simulink model "sm_vehicle_2axle_heave_roll_grid"  (R2024a)
settings: Solver=ode23t  StartTime=0.0  StopTime=14.2  MaxStep=0.2  RelTol=1e-3  AbsTol=1e-3  EnableMultiTasking=on
PostLoadFcn:
  | sm_vehicle_2axle_heave_roll_param
  | sm_vehicle_2axle_heave_roll_scene
  | sm_vehicle_2axle_heave_roll_config_maneuver(bdroot,VehicleData,'rough road');
StartFcn:
  | tic
StopFcn:
  | Elapsed_Sim_Time = toc;
undefined symbols (not defined in the file): InitVehicle, Maneuver, SceneData, VehicleData, X, Y, Z
libraries: sm_lib x48, sm_vehicle_utilities_lib x13, nesl_utility x11
(part 1 of 2)
CloseFcn:
  | try,close(h1_sm_vehicle_2axle_heave_roll),end
  | clear h1_sm_vehicle_2axle_heave_roll
  | try,close(h2_sm_vehicle_2axle_heave_roll),end
  | clear h2_sm_vehicle_2axle_heave_roll
  | try,close(h3_sm_vehicle_2axle_heave_roll),end
  | clear h3_sm_vehicle_2axle_heave_roll
  | 
  | 
  | clear simlog_sm_vehicle_2axle_heave_roll
  | clear logsout_sm_vehicle_2axle_heave_roll
Description:
  | Vehicle Dynamics, 14 DOF Model, Uneven Terrain
  | 
  | Copyright 2022-2024 The MathWorks, Inc.
settings Model: Creator=smiller  LastModifiedBy=smiller
settings SolverCC: AutoScaleAbsTol=off  AlgebraicLoopSolver=TrustRegion
settings DataIOCC: SaveFormat=Array  SaveOutput=off  ReturnWorkspaceOutputs=off  SignalLoggingName=logsout_sm_vehicle_2axle_heave_roll_grid  OutputTimes=[0:0.01:10]
settings OptimizationCC: ReuseModelBlockBuffer=off  ExpressionDepthLimit=2147483647  LifeSpan=inf
settings DebuggingCC: UnderspecifiedInitializationDetection=Classic  MergeDetectMultiDrivingBlocksExec=none  SolverPrmCheckMsg=warning  UnconnectedInputMsg=warning  UnconnectedOutputMsg=warning  UnconnectedLineMsg=warning  StateNameClashWarn=warning  PregeneratedLibrarySubsystemCodeDiagnostic=none  SFUnexpectedBacktrackingDiag=warning  SFNoUnconditionalDefaultTransitionDiag=warning  SFExecutionAtInitializationDiag=none  ArithmeticOperatorsInVariantConditions=warning
settings HardwareCC: ProdBitPerPointer=32  ProdBitPerSizeT=32  ProdBitPerPtrDiffT=32  ProdLargestAtomicFloat=None  ProdIntDivRoundTo=Undefined  ProdEndianess=Unspecified  ProdWordSize=32  ProdHWDeviceType=32-bit Generic
settings ModelReferenceCC: EnableRefExpFcnMdlSchedulingChecks=on  PropagateSignalLabelsOutOfModel=off
settings SFSimCC: SimUseLocalCustomCode=off  CustomCodeUndefinedFunction=UseInterfaceOnly
settings RTWCC: RTWUseLocalCustomCode=off  GPUComputeCapability=3.5  DLArmComputeVersion=19.05
settings CodeAppCC: StateflowObjectComments=on
settings GRTTargetCC: TargetLangStandard=C89/C90 (ANSI)
settings ConfigComp: CovMetricSettings=dw  CovSaveCumulativeToWorkspaceVar=on  CovSaveSingleToWorkspaceVar=on  CovExternalEMLEnable=off
settings SimscapeCC: SimscapeNormalizeSystem=off  SimscapeLogType=all  SimscapeLogToSDI=on  SimscapeLogName=simlog_sm_vehicle_2axle_heave_roll_grid
settings ConfigurationSet: Description=SimMechanics 2G
settings DiagnosticsConfigSet: SimMechanicsUnconnectedFramePorts=none  SimMechanicsConflictingReferenceFrames=none
settings ExplorerConfigSet: InternalSimMechanicsExplorerSettings="<ExplorerConfiguration><canonicalview>default</canonicalview><AnimationSetting><BasePlaybackSpeed>1.0</BasePlaybackSpeed><PlaybackSpeedFactor>2.0</PlaybackSpeedFactor></AnimationSetting><TilePanel><TileInfo><Tiles Columns=\"2\" Count=\"3\" Rows=\"2\"><Column Weight=\"0.6147\"/><Column Weight=\"0.3853\"/><Row Weight=\"0.3693\"/><Row Weight=\"0.6307\"/><Tile Height=\"1\" Width=\"1\" X=\"0\" Y=\"0\"/><Tile Height=\"1\" Width=\"1\" X=\"0\" Y=\"1\"/><Tile Height=\"2\" Width=\"1\" X=\"1\" Y=\"0\"/></Tiles></TileInfo><SceneInfo><SceneViewer><BGColor><R>1</R><G>1</G><B>1</B></BGColor><Camera><DoPerspective>on</DoPerspective><Position><X>-1.49999999999999911</X><Y>1.54074395550978868e-32</Y><Z>10.6999999999999993</Z></Position><Center><X>-1.49999999999999911</X><Y>1.54074395550978868e-32</Y><Z>9.69999999999999929</Z></Center><Up><X>0</X><Y>1</Y><Z>0</Z></Up><ViewLimDist>1</ViewLimDist><YLim>0.466307658154998583</YLim><XLim>1.34838716914770518</XLim></Camera></SceneViewer><SceneViewer><BGColor><R>1</R><G>1</G><B>1</B></BGColor><Camera><DoPerspective>on</DoPerspective><Position><X>2.34000000000000163</X><Y>-3.20000000000000151</Y><Z>1.80000000000000004</Z></Position><Center><X>1.58973091910295716</X><Y>-2.57477576591913149</Y><Z>1.58507916953470085</Z></Center><Up><X>-0.16510675539218278</X><Y>0.137588962826818928</Y><Z>0.976631474319820447</Z></Up><ViewLimDist>1</ViewLimDist><YLim>0.466307658154998583</YLim><XLim>0.779836453951521791</XLim></Camera></SceneViewer><SceneViewer><BGColor><R>1</R><G>1</G><B>1</B></BGColor><Camera><DoPerspective>on</DoPerspective><Position><X>-6.5</X><Y>3.46944695195361419e-16</Y><Z>1.79999999999999982</Z></Position><Center><X>-5.52335553329491002</X><Y>3.46944695195361419e-16</Y><Z>1.58513821732488003</Z></Center><Up><X>0.214861782675119795</X><Y>-1.71056941445900502e-49</Y><Z>0.976644466705089975</Z></Up><ViewLimDist>1</ViewLimDist><YLim>0.466307658154998583</YLim><XLim>0.303969645724483983</XLim></Camera></SceneViewer></SceneInfo></TilePanel><MechEditorPanel><Cameras><Camera><Id>Camera1</Id><Value><Name>Track FixO FR</Name><NativeCamera><PositionTrackingFeature>Vehicle.Camera_Frames.Frame_FixO_FR.R</PositionTrackingFeature><CenterTrackingFeature>Vehicle.Camera_Frames.Frame_FixO_FR.R</CenterTrackingFeature><UpVectorTrackingFeature>Vehicle.Camera_Frames.Frame_FixO_FR.R</UpVectorTrackingFeature><CenterTrackingOrigin>off</CenterTrackingOrigin><CenterTrackingDirection>+X</CenterTrackingDirection><UpVectorTrackingDirection>+Z</UpVectorTrackingDirection></NativeCamera></Value></Camera><Camera><Id>Camera2</Id><Value><Name>Track FixO Right</Name><NativeCamera><PositionTrackingFeature>Vehicle.Camera_Frames.Frame_FixO_Right.R</PositionTrackingFeature><CenterTrackingFeature>Vehicle.Camera_Frames.Frame_FixO_Right.R</CenterTrackingFeature><UpVectorTrackingFeature>Vehicle.Camera_Frames.Frame_FixO_Right.R</UpVectorTrackingFeature><CenterTrackingOrigin>off</CenterTrackingOrigin><CenterTrackingDirection>+X</CenterTrackingDirection><UpVectorTrackingDirection>+Z</UpVectorTrackingDirection></NativeCamera></Value></Camera><Camera><Id>Camera3</Id><Value><Name>Track FixO RR</Name><NativeCamera><PositionTrackingFeature>Vehicle.Camera_Frames.Frame_FixO_RR.R</PositionTrackingFeature><CenterTrackingFeature>Vehicle.Camera_Frames.Frame_FixO_RR.R</CenterTrackingFeature><UpVectorTrackingFeature>Vehicle.Camera_Frames.Frame_FixO_RR.R</UpVectorTrackingFeature><CenterTrackingOrigin>off</CenterTrackingOrigin><CenterTrackingDirection>+X</CenterTrackingDirection><UpVectorTrackingDirection>+Z</UpVectorTrackingDirection></NativeCamera></Value></Camera><Camera><Id>Camera4</Id><Value><Name>Track FixO RL</Name><NativeCamera><PositionTrackingFeature>Vehicle.Camera_Frames.Frame_FixO_RL.R</PositionTrackingFeature><CenterTrackingFeature>Vehicle.Camera_Frames.Frame_FixO_RL.R</CenterTrackingFeature><UpVectorTrackingFeature>Vehicle.Camera_Frames.Frame_FixO_RL.R</UpVectorTrackingFeature><CenterTrackingOrigin>off</CenterTrackingOrigin><CenterTrackingDirection>+X</CenterTrackingDirection><UpVectorTrackingDirection>+Z</UpVectorTrackingDirection></NativeCamera></Value></Camera><Camera><Id>Camera5</Id><Value><Name>Track FixO Left</Name><NativeCamera><PositionTrackingFeature>Vehicle.Camera_Frames.Frame_FixO_Left.R</PositionTrackingFeature><CenterTrackingFeature>Vehicle.Camera_Frames.Frame_FixO_Left.R</CenterTrackingFeature><UpVectorTrackingFeature>Vehicle.Camera_Frames.Frame_FixO_Left.R</UpVectorTrackingFeature><CenterTrackingOrigin>off</CenterTrackingOrigin><CenterTrackingDirection>+X</CenterTrackingDirection><UpVectorTrackingDirection>+Z</UpVectorTrackingDirection></NativeCamera></Value></Camera><Camera><Id>Camera6</Id><Value><Name>Track FixO FL</Name><NativeCamera><PositionTrackingFeature>Vehicle.Camera_Frames.Frame_FixO_FL.R</PositionTrackingFeature><CenterTrackingFeature>Vehicle.Camera_Frames.Frame_FixO_FL.R</CenterTrackingFeature><UpVectorTrackingFeature>Vehicle.Camera_Frames.Frame_FixO_FL.R</UpVectorTrackingFeature><CenterTrackingOrigin>off</CenterTrackingOrigin><CenterTrackingDirection>+X</CenterTrackingDirection><UpVectorTrackingDirection>+Z</UpVectorTrackingDirection></NativeCamera></Value></Camera><Camera><Id>Camera7</Id><Value><Name>Track FixO Top</Name><NativeCamera><PositionTrackingFeature>Vehicle.Camera_Frames.Frame_FixO_Top.R</PositionTrackingFeature><CenterTrackingFeature>Vehicle.Camera_Frames.Frame_FixO_Top.R</CenterTrackingFeature><UpVectorTrackingFeature>Vehicle.Camera_Frames.Frame_FixO_Top.R</UpVectorTrackingFeature><CenterTrackingOrigin>off</CenterTrackingOrigin><CenterTrackingDirection>+X</CenterTrackingDirection><UpVectorTrackingDirection>+Z</UpVectorTrackingDirection></NativeCamera></Value></Camera><Camera><Id>Camera8</Id><Value><Name>Track FixO Front</Name><NativeCamera><PositionTrackingFeature>Vehicle.Camera_Frames.Frame_FixO_Front.R</PositionTrackingFeature><CenterTrackingFeature>Vehicle.Camera_Frames.Frame_FixO_Front.R</CenterTrackingFeature><UpVectorTrackingFeature>Vehicle.Camera_Frames.Frame_FixO_Front.R</UpVectorTrackingFeature><CenterTrackingOrigin>off</CenterTrackingOrigin><CenterTrackingDirection>+X</CenterTrackingDirection><UpVectorTrackingDirection>+Z</UpVectorTrackingDirection></NativeCamera></Value></Camera><Camera><Id>Camera9</Id><Value><Name>Track FixO Rear</Name><NativeCamera><PositionTrackingFeature>Vehicle.Camera_Frames.Frame_FixO_Rear.R</PositionTrackingFeature><CenterTrackingFeature>Vehicle.Camera_Frames.Frame_FixO_Rear.R</CenterTrackingFeature><UpVectorTrackingFeature>Vehicle.Camera_Frames.Frame_FixO_Rear.R</UpVectorTrackingFeature><CenterTrackingOrigin>off</CenterTrackingOrigin><CenterTrackingDirection>+X</CenterTrackingDirection><UpVectorTrackingDirection>+Z</UpVectorTrackingDirection></NativeCamera></Value></Camera><Camera><Id>Camera10</Id><Value><Name>Track FR</Name><NativeCamera><PositionTrackingFeature>Vehicle.Camera_Frames.Frame_FR.R</PositionTrackingFeature><CenterTrackingFeature>Vehicle.Camera_Frames.Frame_FR.R</CenterTrackingFeature><UpVectorTrackingFeature>Vehicle.Camera_Frames.Frame_FR.R</UpVectorTrackingFeature><CenterTrackingOrigin>off</CenterTrackingOrigin><CenterTrackingDirection>+X</CenterTrackingDirection><UpVectorTrackingDirection>+Z</UpVectorTrackingDirection></NativeCamera></Value></Camera><Camera><Id>Camera11</Id><Value><Name>Track Right</Name><NativeCamera><PositionTrackingFeature>Vehicle.Camera_Frames.Frame_Right.R</PositionTrackingFeature><CenterTrackingFeature>Vehicle.Camera_Frames.Frame_Right.R</CenterTrackingFeature><UpVectorTrackingFeature>Vehicle.Camera_Frames.Frame_Right.R</UpVectorTrackingFeature><CenterTrackingOrigin>off</CenterTrackingOrigin><CenterTrackingDirection>+X</CenterTrackingDirection><UpVectorTrackingDirection>+Z</UpVectorTrackingDirection></NativeCamera></Value></Camera><Camera><Id>Camera12</Id><Value><Name>Track RR</Name><NativeCamera><PositionTrackingFeature>Vehicle.Camera_Frames.Frame_RR.R</PositionTrackingFeature><CenterTrackingFeature>Vehicle.Camera_Frames.Frame_RR.R</CenterTrackingFeature><UpVectorTrackingFeature>Vehicle.Camera_Frames.Frame_RR.R</UpVectorTrackingFeature><CenterTrackingOrigin>off</CenterTrackingOrigin><CenterTrackingDirection>+X</CenterTrackingDirection><UpVectorTrackingDirection>+Z</UpVectorTrackingDirection></NativeCamera></Value></Camera><Camera><Id>Camera13</Id><Value><Name>Track RL</Name><NativeCamera><PositionTrackingFeature>Vehicle.Camera_Frames.Frame_RL.R</PositionTrackingFeature><CenterTrackingFeature>Vehicle.Camera_Frames.Frame_RL.R</CenterTrackingFeature><UpVectorTrackingFeature>Vehicle.Camera_Frames.Frame_RL.R</UpVectorTrackingFeature><CenterTrackingOrigin>off</CenterTrackingOrigin><CenterTrackingDirection>+X</CenterTrackingDirection><UpVectorTrackingDirection>+Z</UpVectorTrackingDirection></NativeCamera></Value></Camera><Camera><Id>Camera14</Id><Value><Name>Track Left</Name><NativeCamera><PositionTrackingFeature>Vehicle.Camera_Frames.Frame_Left.R</PositionTrackingFeature><CenterTrackingFeature>Vehicle.Camera_Frames.Frame_Left.R</CenterTrackingFeature><UpVectorTrackingFeature>Vehicle.Camera_Frames.Frame_Left.R</UpVectorTrackingFeature><CenterTrackingOrigin>off</CenterTrackingOrigin><CenterTrackingDirection>+X</CenterTrackingDirection><UpVectorTrackingDirection>+Z</UpVectorTrackingDirection></NativeCamera></Value></Camera><Camera><Id>Camera15</Id><Value><Name>Track FL</Name><NativeCamera><PositionTrackingFeature>Vehicle.Camera_Frames.Frame_FL.R</PositionTrackingFeature><CenterTrackingFeature>Vehicle.Camera_Frames.Frame_FL.R</CenterTrackingFeature><UpVectorTrackingFeature>Vehicle.Camera_Frames.Frame_FL.R</UpVectorTrackingFeature><CenterTrackingOrigin>off</CenterTrackingOrigin><CenterTrackingDirection>+X</CenterTrackingDirection><UpVectorTrackingDirection>+Z</UpVectorTrackingDirection></NativeCamera></Value></Camera><Camera><Id>Camera16</Id><Value><Name>Track Top</Name><NativeCamera><PositionTrackingFeature>Vehicle.Camera_Frames.Frame_Top.R</PositionTrackingFeature><CenterTrackingFeature>Vehicle.Camera_Frames.Frame_Top.R</CenterTrackingFeature><UpVectorTrackingFeature>Vehicle.Camera_Frames.Frame_Top.R</UpVectorTrackingFeature><CenterTrackingOrigin>off</CenterTrackingOrigin><CenterTrackingDirection>+X</CenterTrackingDirection><UpVectorTrackingDirection>+Z</UpVectorTrackingDirection></NativeCamera></Value></Camera><Camera><Id>Camera17</Id><Value><Name>Track Front</Name><NativeCamera><PositionTrackingFeature>Vehicle.Camera_Frames.Frame_Front.R</PositionTrackingFeature><CenterTrackingFeature>Vehicle.Camera_Frames.Frame_Front.R</CenterTrackingFeature><UpVectorTrackingFeature>Vehicle.Camera_Frames.Frame_Front.R</UpVectorTrackingFeature><CenterTrackingOrigin>off</CenterTrackingOrigin><CenterTrackingDirection>+X</CenterTrackingDirection><UpVectorTrackingDirection>+Z</UpVectorTrackingDirection></NativeCamera></Value></Camera><Camera><Id>Camera18</Id><Value><Name>Track Rear</Name><NativeCamera><PositionTrackingFeature>Vehicle.Camera_Frames.Frame_Rear.R</PositionTrackingFeature><CenterTrackingFeature>Vehicle.Camera_Frames.Frame_Rear.R</CenterTrackingFeature><UpVectorTrackingFeature>Vehicle.Camera_Frames.Frame_Rear.R</UpVectorTrackingFeature><CenterTrackingOrigin>off</CenterTrackingOrigin><CenterTrackingDirection>+X</CenterTrackingDirection><UpVectorTrackingDirection>+Z</UpVectorTrackingDirection></NativeCamera></Value></Camera><Camera><Id>Camera19</Id><Value><Name>Track SuspF</Name><NativeCamera><PositionTrackingFeature>Vehicle.Camera_Frames.Frame_SuspF.R</PositionTrackingFeature><CenterTrackingFeature>Vehicle.Camera_Frames.Frame_SuspF.R</CenterTrackingFeature><UpVectorTrackingFeature>Vehicle.Camera_Frames.Frame_SuspF.R</UpVectorTrackingFeature><CenterTrackingOrigin>off</CenterTrackingOrigin><CenterTrackingDirection>+X</CenterTrackingDirection><UpVectorTrackingDirection>+Z</UpVectorTrackingDirection></NativeCamera></Value></Camera><Camera><Id>Camera20</Id><Value><Name>Track SuspR</Name><NativeCamera><PositionTrackingFeature>Vehicle.Camera_Frames.Frame_SuspR.R</PositionTrackingFeature><CenterTrackingFeature>Vehicle.Camera_Frames.Frame_SuspR.R</CenterTrackingFeature><UpVectorTrackingFeature>Vehicle.Camera_Frames.Frame_SuspR.R</UpVectorTrackingFeature><CenterTrackingOrigin>off</CenterTrackingOrigin><CenterTrackingDirection>+X</CenterTrackingDirection><UpVectorTrackingDirection>+Z</UpVectorTrackingDirection></NativeCamera></Value></Camera><Camera><Id>Camera21</Id><Value><Name>Track WheelFR</Name><NativeCamera><PositionTrackingFeature>Vehicle.Camera_Frames.Frame_Wheel_FR.R</PositionTrackingFeature><CenterTrackingFeature>Vehicle.Camera_Frames.Frame_Wheel_FR.R</CenterTrackingFeature><UpVectorTrackingFeature>Vehicle.Camera_Frames.Frame_Wheel_FR.R</UpVectorTrackingFeature><CenterTrackingOrigin>off</CenterTrackingOrigin><CenterTrackingDirection>+X</CenterTrackingDirection><UpVectorTrackingDirection>+Z</UpVectorTrackingDirection></NativeCamera></Value></Camera><Camera><Id>Camera22</Id><Value><Name>Track WheelRR</Name><NativeCamera><PositionTrackingFeature>Vehicle.Camera_Frames.Frame_Wheel_RR.R</PositionTrackingFeature><CenterTrackingFeature>Vehicle.Camera_Frames.Frame_Wheel_RR.R</CenterTrackingFeature><UpVectorTrackingFeature>Vehicle.Camera_Frames.Frame_Wheel_RR.R</UpVectorTrackingFeature><CenterTrackingOrigin>off</CenterTrackingOrigin><CenterTrackingDirection>+X</CenterTrackingDirection><UpVectorTrackingDirection>+Z</UpVectorTrackingDirection></NativeCamera></Value></Camera><Camera><Id>Camera23</Id><Value><Name>Track WheelRL</Name><NativeCamera><PositionTrackingFeature>Vehicle.Camera_Frames.Frame_Wheel_RL.R</PositionTrackingFeature><CenterTrackingFeature>Vehicle.Camera_Frames.Frame_Wheel_RL.R</CenterTrackingFeature><UpVectorTrackingFeature>Vehicle.Camera_Frames.Frame_Wheel_RL.R</UpVectorTrackingFeature><CenterTrackingOrigin>off</CenterTrackingOrigin><CenterTrackingDirection>+X</CenterTrackingDirection><UpVectorTrackingDirection>+Z</UpVectorTrackingDirection></NativeCamera></Value></Camera><Camera><Id>Camera24</Id><Value><Name>Track WheelFL</Name><NativeCamera><PositionTrackingFeature>Vehicle.Camera_Frames.Frame_Wheel_FL.R</PositionTrackingFeature><CenterTrackingFeature>Vehicle.Camera_Frames.Frame_Wheel_FL.R</CenterTrackingFeature><UpVectorTrackingFeature>Vehicle.Camera_Frames.Frame_Wheel_FL.R</UpVectorTrackingFeature><CenterTrackingOrigin>off</CenterTrackingOrigin><CenterTrackingDirection>+X</CenterTrackingDirection><UpVectorTrackingDirection>+Z</UpVectorTrackingDirection></NativeCamera></Value></Camera><Camera><Id>Camera25</Id><Value><Name>View Seat FL</Name><NativeCamera><PositionTrackingFeature>Vehicle.Camera_Frames.Frame_View_Seat_FL.R</PositionTrackingFeature><CenterTrackingFeature>Vehicle.Camera_Frames.Frame_View_Seat_FL.R</CenterTrackingFeature><UpVectorTrackingFeature>Vehicle.Camera_Frames.Frame_View_Seat_FL.R</UpVectorTrackingFeature><CenterTrackingOrigin>off</CenterTrackingOrigin><CenterTrackingDirection>+X</CenterTrackingDirection><UpVectorTrackingDirection>+Z</UpVectorTrackingDirection></NativeCamera></Value></Camera><Camera><Id>Camera26</Id><Value><Name>View Seat FR</Name><NativeCamera><PositionTrackingFeature>Vehicle.Camera_Frames.Frame_View_Seat_FR.R</PositionTrackingFeature><CenterTrackingFeature>Vehicle.Camera_Frames.Frame_View_Seat_FR.R</CenterTrackingFeature><UpVectorTrackingFeature>Vehicle.Camera_Frames.Frame_View_Seat_FR.R</UpVectorTrackingFeature><CenterTrackingOrigin>off</CenterTrackingOrigin><CenterTrackingDirection>+X</CenterTrackingDirection><UpVectorTrackingDirection>+Z</UpVectorTrackingDirection></NativeCamera></Value></Camera><Camera><Id>Camera27</Id><Value><Name>View Susp FR</Name><NativeCamera><PositionTrackingFeature>Vehicle.Camera_Frames.Frame_View_Susp_FR.R</PositionTrackingFeature><CenterTrackingFeature>Vehicle.Camera_Frames.Frame_View_Susp_FR.R</CenterTrackingFeature><UpVectorTrackingFeature>Vehicle.Camera_Frames.Frame_View_Susp_FR.R</UpVectorTrackingFeature><CenterTrackingOrigin>off</CenterTrackingOrigin><CenterTrackingDirection>+X</CenterTrackingDirection><UpVectorTrackingDirection>+Z</UpVectorTrackingDirection></NativeCamera></Value></Camera><Camera><Id>Camera28</Id><Value><Name>View Susp RR</Name><NativeCamera><PositionTrackingFeature>Vehicle.Camera_Frames.Frame_View_Susp_RR.R</PositionTrackingFeature><CenterTrackingFeature>Vehicle.Camera_Frames.Frame_View_Susp_RR.R</CenterTrackingFeature><UpVectorTrackingFeature>Vehicle.Camera_Frames.Frame_View_Susp_RR.R</UpVectorTrackingFeature><CenterTrackingOrigin>off</CenterTrackingOrigin><CenterTrackingDirection>+X</CenterTrackingDirection><UpVectorTrackingDirection>+Z</UpVectorTrackingDirection></NativeCamera></Value></Camera><Camera><Id>Camera29</Id><Value><Name>View Susp RL</Name><NativeCamera><PositionTrackingFeature>Vehicle.Camera_Frames.Frame_View_Susp_RL.R</PositionTrackingFeature><CenterTrackingFeature>Vehicle.Camera_Frames.Frame_View_Susp_RL.R</CenterTrackingFeature><UpVectorTrackingFeature>Vehicle.Camera_Frames.Frame_View_Susp_RL.R</UpVectorTrackingFeature><CenterTrackingOrigin>off</CenterTrackingOrigin><CenterTrackingDirection>+X</CenterTrackingDirection><UpVectorTrackingDirection>+Z</UpVectorTrackingDirection></NativeCamera></Value></Camera><Camera><Id>Camera30</Id><Value><Name>View Susp FL</Name><NativeCamera><PositionTrackingFeature>Vehicle.Camera_Frames.Frame_View_Susp_FL.R</PositionTrackingFeature><CenterTrackingFeature>Vehicle.Camera_Frames.Frame_View_Susp_FL.R</CenterTrackingFeature><UpVectorTrackingFeature>Vehicle.Camera_Frames.Frame_View_Susp_FL.R</UpVectorTrackingFeature><CenterTrackingOrigin>off</CenterTrackingOrigin><CenterTrackingDirection>+X</CenterTrackingDirection><UpVectorTrackingDirection>+Z</UpVectorTrackingDirection></NativeCamera></Value></Camera><Camera><Id>Camera31</Id><Value><Name>Dolly Camera</Name><NativeCamera><PositionTrackingFeature>Vehicle.Camera_Frames.Frame_Dolly.R</PositionTrackingFeature><CenterTrackingFeature>Vehicle.Camera_Frames.Frame_Dolly.R</CenterTrackingFeature><UpVectorTrackingFeature>Vehicle.Camera_Frames.Frame_Dolly.R</UpVectorTrackingFeature><CenterTrackingOrigin>off</CenterTrackingOrigin><CenterTrackingDirection>+X</CenterTrackingDirection><UpVectorTrackingDirection>+Z</UpVectorTrackingDirection></NativeCamera></Value></Camera><Camera><Id>Camera32</Id><Value><Name>Track Dolly Camera</Name><NativeCamera><PositionTrackingFeature>Vehicle.Camera_Frames.Frame_Dolly.R</PositionTrackingFeature><CenterTrackingFeature>Vehicle.Camera_Frames.Transform_Camera_Ref.F</CenterTrackingFeature><UpVectorTrackingFeature>Vehicle.Camera_Frames.World_Frame.W</UpVectorTrackingFeature><CenterTrackingOrigin>on</CenterTrackingOrigin><UpVectorTrackingDirection>+Z</UpVectorTrackingDirection></NativeCamera></Value></Camera></Cameras><GfxPanelCameraMap><MapElement CameraMLId=\"Camera7\" GfxPanelIndex=\"0\"/><MapElement CameraMLId=\"Camera1\" GfxPanelIndex=\"1\"/><MapElement CameraMLId=\"Camera9\" GfxPanelIndex=\"2\"/></GfxPanelCameraMap><VideoCreator><PlaybackSpeedRatio>1.0</PlaybackSpeedRatio><FrameRate>30</FrameRate><VideoFormat>MPEG-4</VideoFormat><FrameSize>[800 450]</FrameSize></VideoCreator></MechEditorPanel></ExplorerConfiguration>"

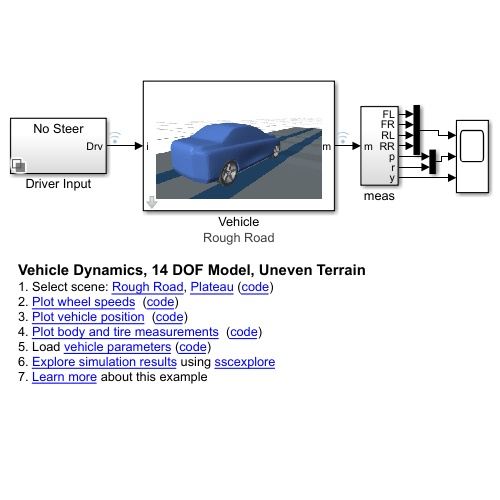
[thumbnail: Simulink's stored preview of the top-level diagram]
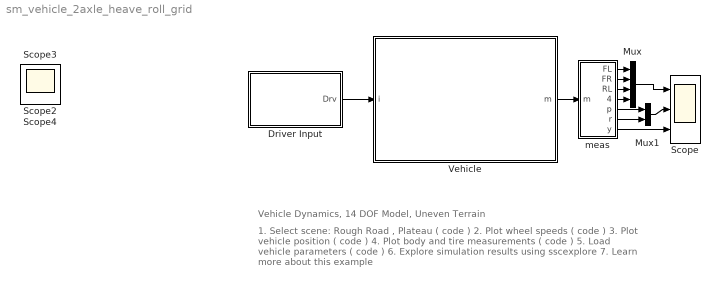
== system sm_vehicle_2axle_heave_roll_grid ==
  note: Vehicle Dynamics, 14 DOF Model, Uneven Terrain
  note: 1. Select scene: Rough Road , Plateau ( code )
      | 2. Plot wheel speeds ( code )
      | 3. Plot vehicle position ( code )
      | 4. Plot body and tire measurements ( code )
      | 5. Load vehicle parameters ( code )
      | 6. Explore simulation results using sscexplore
      | 7. Learn more about this example
  Driver Input : Subsystem  Variant=on  VariantControlMode=label  LabelModeActiveChoice=NoSteer
  Mux : Mux
  Mux1 : Mux  Inputs=2
  Scope : Scope  NumInputPorts=3
  Vehicle : Subsystem  mask(Vehicle and Scene){vehdata=VehicleData, initveh=InitVehicle, popup_scene=Rough Road}
      mask prompts: vehdata "Vehicle Data (structure)"; initveh "Initial Position, Velocity (structure)"; popup_scene "Scene"
      mask help: Models a vehicle with a configurable scene. Vehicle parameters are defined within a single data structure. A separate data structure defines the initial position, orientation, and speed of the vehicle and the wheels.
      mask init:
      | scene_name = strrep(get_param(gcb,'popup_scene'),' ','_');
      | set_param([gcb '/Scene'],'LabelModeActiveChoice',scene_name);
      | switch(scene_name)
      |     case('Plateau')
      |         Plateau = evalin('base','SceneData.Plateau');
      |         grid_surf_x = Plateau.Road.pzLUT.px;
      |         grid_surf_y = [-4  4];
      |         grid_surf_z = Plateau.Road.pzLUT.pz;
      |     case('Rough_Road')
      |         Rough_Road = evalin('base','SceneData.Rough_Road');
      |         grid_surf_x = Rough_Road.Road.pzLUT.px;
      |         grid_surf_y = [-4  -0.5 0 0.5 4];
      |         grid_surf_z = [...
      |             Rough_Road.Road.pzLUT.pz(:,2) ...
      |             Rough_Road.Road.pzLUT.pz(:,2) ...
      |             sum(Rough_Road.Road.pzLUT.pz,2)/2 ...
      |             Rough_Road.Road.pzLUT.pz(:,1) ...
      |             Rough_Road.Road.pzLUT.pz(:,1)];
      | end
      settings: AttributesFormatString=%<popup_scene>
      mask TypeOptions popup_scene: Plateau | Rough Road
      mask Display:
      | scene_name = lower(strrep(get_param(gcb,'popup_scene'),' ','_'));
      | image(['sm_vehicle_2axle_heave_roll_vehicle_grid_' scene_name '.png']);
      | % Notes for mask images
      | % Screenshot taken MechExp 931x463, one pane 619x314
      | % Trim to 434 x 272, resize to 500x330
  meas : Subsystem
  Scope2 : Scope
  Scope3 : Scope
  Scope4 : Scope
  wires:
  Driver Input/1(Drv) -> Vehicle/1(i)
  Vehicle/1(m) -> meas/1(m)
  Mux/1 -> Scope/1
  meas/1(FL) -> Mux/1
  meas/2(FR) -> Mux/2
  meas/3(RL) -> Mux/3
  meas/4(RR) -> Mux/4
  meas/5(p) -> Mux1/1
  meas/6(r) -> Mux1/2
  Mux1/1 -> Scope/2
  meas/7(y) -> Scope/3

== system sm_vehicle_2axle_heave_roll_grid/Driver Input ==
  No Steer : Subsystem  VariantControl=NoSteer
  Parking : Subsystem  VariantControl=Parking
  Sine With Dwell : Subsystem  VariantControl=SineWithDwell
  Slalom : Subsystem  VariantControl=Slalom
  Step Steer : Subsystem  VariantControl=StepSteer
  Drv : Outport

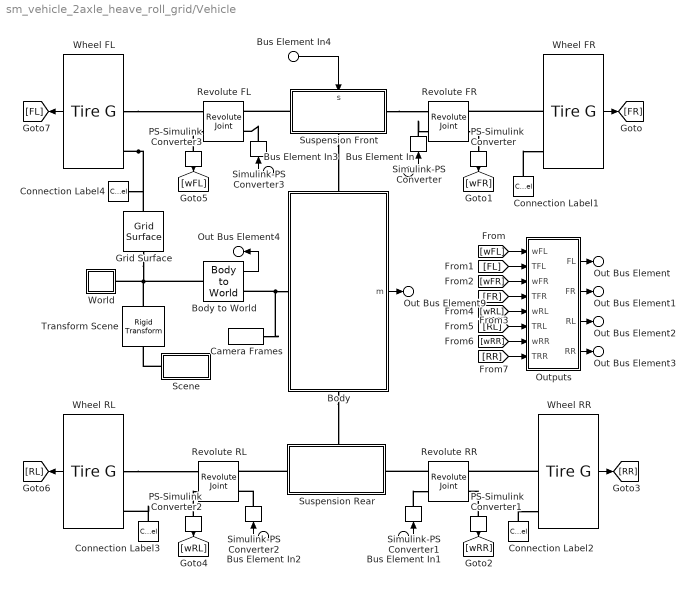
== system sm_vehicle_2axle_heave_roll_grid/Vehicle ==
  Bus Element In : Inport  PortName=i  Element=trqFR
  Bus Element In1 : Inport  PortName=i  Element=trqRR
  Bus Element In2 : Inport  PortName=i  Element=trqRL
  Bus Element In3 : Inport  PortName=i  Element=trqFL
  Bus Element In4 : Inport  PortName=i  Element=sWhl
  Body : Subsystem  mask(Body for 2-Axle Vehicle){xRefToFA=vehdata.Body.FA, xRefToRA=vehdata.Body.RA, xyzRefToCG=vehdata.Body.CG, xyzRefToGeometry=vehdata.Body.Geometry, mBody=vehdata.Body.Mass, JBody=vehdata.Body.Inertias, clrBody=vehdata.Body.Color, opcBody=vehdata.Body.Opacity}
      mask prompts: xRefToFA "Offset Reference to Front Axle (m)"; xRefToRA "Offset Reference to Rear Axle (m)"; xyzRefToCG "Offset Reference to CG [x y z] (m)"; xyzRefToGeometry "Offset Reference to Geometry [x y z] (m)"; mBody "Body Mass (kg)"; JBody "Body Inertia [Ixx Iyy Izz] (kg*m^2)"; clrBody "Body Color [R G B]"; opcBody "Body Opacity (0-1)"
      mask help: Models mass and inertia of rigid vehicle body. Frames for front suspension, rear suspension, center of gravity, and body geometry are all defined relative to the reference frame. Measurements are with respect to the body frame.
      settings: PortSchema="{\"entries\":[{\"content\":{\"sides\":[{\"content\":{\"connectorIds\":[\"LConn1\"]},\"type\":\"ConnectorPlacement.EquallySpacedRectSide\",\"uuid\":\"a6a40084-0b01-416d-a19a-d775fde84bbf\"},{\"content\":{\"connectorIds\":[\"RConn1\"],\"side\":\"RIGHT\"},\"type\":\"ConnectorPlacement.EquallySpacedRectSide\",\"uuid\":\"7b527776-1265-46e3-b587-d37cab880183\"},{\"content\":{\"connectorIds\":[\"Out1\"],\"side\":\"TOP\"},\"type\":\"ConnectorPlacement.EquallySpacedRectSide\",\"uuid\":\"f01e2205-af4e-42ab-b4af-31b005ea0e61\"},{\"content\":{\"connectorIds\":[\"RConn2\"],\"side\":\"BOTTOM\"},\"type\":\"ConnectorPlacement.EquallySpacedRectSide\",\"uuid\":\"682a6e2c-9f3d-4bbb-bb88-e5eb72c2e6bf\"}]},\"type\":\"ConnectorPlacement.EquallySpacedConnector\",\"uuid\":\"a1282978-4c55-459b-9a00-856109b4503f\"}],\"packageUris\":[\"http://schema.mathworks.com/mf0/Connector/R2020b\"],\"version\":\"1.0\"}"
      mask Display: image('sm_vehicle_utilities_body_sedan.png');
  Body to World : sm_vehicle_utilities_lib/Body to World  Init=initveh.Vehicle  SpecifyPosTarget=on
  Camera Frames : sm_vehicle_utilities_lib/Camera Frames  Camera=Camera  popup_dolly_camera=Off
  Connection Label{1..4} (4 alike) : ConnectionLabel  Label=Terrain
  Grid Surface : sm_lib/Curves and Surfaces/Grid Surface  XGridVector=grid_surf_x  XGridVectorUnits=m  YGridVector=grid_surf_y  YGridVectorUnits=m  ZHeights=grid_surf_z  ZHeightsUnits=m  GraphicType=FromGeometry  GraphicVisPropType=AdvancedVisualProperties  GraphicDiffuseColor=[0.4549 0.5451 0.5882]  GraphicOpacity=1.0  GraphicSpecularColor=[0.9 0.9 0.9 01]  GraphicAmbientColor=[0.25 0.25 0.25 1.0]  GraphicEmissiveColor=[0.0 0.0 0.0 1.0]  GraphicShininess=75
  Outputs : Subsystem
  PS-Simulink Converter{,1..3} (4 alike) : nesl_utility/PS-Simulink Converter  PhysicalDomain=network_engine_domain  SubClassName=ps_output  LeftPortType=input  RightPortType=output  PseudoPeriodic=off  Frequencies=[]  VectorFormat=1-D array  Unit=inherit  AffineConversion=off
  Revolute FL : sm_lib/Joints/Revolute Joint  JointMode=Normal  CompositeWrenchDir=FollowerOnBase  CompositeWrenchFrame=BaseFrame  SenseConstraintForce=off  SenseConstraintTorque=off  SenseTotalForce=off  SenseTotalTorque=off  PositionTargetSpecify=off  PositionTargetPriority=High  PositionTargetValue=0  PositionTargetValueUnits=deg  VelocityTargetSpecify=on  VelocityTargetPriority=High  VelocityTargetValue=initveh.Wheel.wFL  VelocityTargetValueUnits=rad/s  EquilibriumPosition=0  EquilibriumPositionUnits=rad  SpringStiffness=0  SpringStiffnessUnits=N*m/rad  DampingCoefficient=0  DampingCoefficientUnits=N*m/(rad/s)  LowerLimitSpecify=off  LowerLimitBound=-90  LowerLimitBoundUnits=deg  LowerLimitStiffness=1e4  LowerLimitStiffnessUnits=N*m/deg  LowerLimitDamping=10  LowerLimitDampingUnits=N*m/(deg/s)  LowerLimitTransitionRegionWidth=0.1  LowerLimitTransitionRegionWidthUnits=deg  UpperLimitSpecify=off  UpperLimitBound=90  UpperLimitBoundUnits=deg  UpperLimitStiffness=1e4  UpperLimitStiffnessUnits=N*m/deg  UpperLimitDamping=10  UpperLimitDampingUnits=N*m/(deg/s)  UpperLimitTransitionRegionWidth=0.1  UpperLimitTransitionRegionWidthUnits=deg  TorqueActuationMode=InputTorque  MotionActuationMode=ComputedMotion  SensePosition=off  SenseVelocity=on  SenseAcceleration=off  SenseTorqueForce=off  SenseLowerLimitTorqueForce=off  SenseUpperLimitTorqueForce=off
  Revolute FR : sm_lib/Joints/Revolute Joint  JointMode=Normal  CompositeWrenchDir=FollowerOnBase  CompositeWrenchFrame=BaseFrame  SenseConstraintForce=off  SenseConstraintTorque=off  SenseTotalForce=off  SenseTotalTorque=off  PositionTargetSpecify=off  PositionTargetPriority=High  PositionTargetValue=0  PositionTargetValueUnits=deg  VelocityTargetSpecify=on  VelocityTargetPriority=High  VelocityTargetValue=initveh.Wheel.wFR  VelocityTargetValueUnits=rad/s  EquilibriumPosition=0  EquilibriumPositionUnits=rad  SpringStiffness=0  SpringStiffnessUnits=N*m/rad  DampingCoefficient=0  DampingCoefficientUnits=N*m/(rad/s)  LowerLimitSpecify=off  LowerLimitBound=-90  LowerLimitBoundUnits=deg  LowerLimitStiffness=1e4  LowerLimitStiffnessUnits=N*m/deg  LowerLimitDamping=10  LowerLimitDampingUnits=N*m/(deg/s)  LowerLimitTransitionRegionWidth=0.1  LowerLimitTransitionRegionWidthUnits=deg  UpperLimitSpecify=off  UpperLimitBound=90  UpperLimitBoundUnits=deg  UpperLimitStiffness=1e4  UpperLimitStiffnessUnits=N*m/deg  UpperLimitDamping=10  UpperLimitDampingUnits=N*m/(deg/s)  UpperLimitTransitionRegionWidth=0.1  UpperLimitTransitionRegionWidthUnits=deg  TorqueActuationMode=InputTorque  MotionActuationMode=ComputedMotion  SensePosition=off  SenseVelocity=on  SenseAcceleration=off  SenseTorqueForce=off  SenseLowerLimitTorqueForce=off  SenseUpperLimitTorqueForce=off
  Revolute RL : sm_lib/Joints/Revolute Joint  JointMode=Normal  CompositeWrenchDir=FollowerOnBase  CompositeWrenchFrame=BaseFrame  SenseConstraintForce=off  SenseConstraintTorque=off  SenseTotalForce=off  SenseTotalTorque=off  PositionTargetSpecify=off  PositionTargetPriority=High  PositionTargetValue=0  PositionTargetValueUnits=deg  VelocityTargetSpecify=on  VelocityTargetPriority=High  VelocityTargetValue=initveh.Wheel.wRL  VelocityTargetValueUnits=rad/s  EquilibriumPosition=0  EquilibriumPositionUnits=rad  SpringStiffness=0  SpringStiffnessUnits=N*m/rad  DampingCoefficient=0  DampingCoefficientUnits=N*m/(rad/s)  LowerLimitSpecify=off  LowerLimitBound=-90  LowerLimitBoundUnits=deg  LowerLimitStiffness=1e4  LowerLimitStiffnessUnits=N*m/deg  LowerLimitDamping=10  LowerLimitDampingUnits=N*m/(deg/s)  LowerLimitTransitionRegionWidth=0.1  LowerLimitTransitionRegionWidthUnits=deg  UpperLimitSpecify=off  UpperLimitBound=90  UpperLimitBoundUnits=deg  UpperLimitStiffness=1e4  UpperLimitStiffnessUnits=N*m/deg  UpperLimitDamping=10  UpperLimitDampingUnits=N*m/(deg/s)  UpperLimitTransitionRegionWidth=0.1  UpperLimitTransitionRegionWidthUnits=deg  TorqueActuationMode=InputTorque  MotionActuationMode=ComputedMotion  SensePosition=off  SenseVelocity=on  SenseAcceleration=off  SenseTorqueForce=off  SenseLowerLimitTorqueForce=off  SenseUpperLimitTorqueForce=off
  Revolute RR : sm_lib/Joints/Revolute Joint  JointMode=Normal  CompositeWrenchDir=FollowerOnBase  CompositeWrenchFrame=BaseFrame  SenseConstraintForce=off  SenseConstraintTorque=off  SenseTotalForce=off  SenseTotalTorque=off  PositionTargetSpecify=off  PositionTargetPriority=High  PositionTargetValue=0  PositionTargetValueUnits=deg  VelocityTargetSpecify=on  VelocityTargetPriority=High  VelocityTargetValue=initveh.Wheel.wRR  VelocityTargetValueUnits=rad/s  EquilibriumPosition=0  EquilibriumPositionUnits=rad  SpringStiffness=0  SpringStiffnessUnits=N*m/rad  DampingCoefficient=0  DampingCoefficientUnits=N*m/(rad/s)  LowerLimitSpecify=off  LowerLimitBound=-90  LowerLimitBoundUnits=deg  LowerLimitStiffness=1e4  LowerLimitStiffnessUnits=N*m/deg  LowerLimitDamping=10  LowerLimitDampingUnits=N*m/(deg/s)  LowerLimitTransitionRegionWidth=0.1  LowerLimitTransitionRegionWidthUnits=deg  UpperLimitSpecify=off  UpperLimitBound=90  UpperLimitBoundUnits=deg  UpperLimitStiffness=1e4  UpperLimitStiffnessUnits=N*m/deg  UpperLimitDamping=10  UpperLimitDampingUnits=N*m/(deg/s)  UpperLimitTransitionRegionWidth=0.1  UpperLimitTransitionRegionWidthUnits=deg  TorqueActuationMode=InputTorque  MotionActuationMode=ComputedMotion  SensePosition=off  SenseVelocity=on  SenseAcceleration=off  SenseTorqueForce=off  SenseLowerLimitTorqueForce=off  SenseUpperLimitTorqueForce=off
  Scene : Subsystem  Variant=on  VariantControlMode=label  LabelModeActiveChoice=Rough_Road
      settings: AttributesFormatString=%<LabelModeActiveChoice>
      mask Display: disp(' ');
  Simulink-PS Converter{,1..3} (4 alike) : nesl_utility/Simulink-PS Converter  PhysicalDomain=network_engine_domain  SubClassName=ps_input  LeftPortType=input  RightPortType=output  PseudoPeriodic=off  Frequencies=[]  NoiseDistribution=none  NoiseParameters=[]  Unit=N*m  AffineConversion=off  FilteringAndDerivatives=provide  SimscapeFilterOrder=1  InputFilterTimeConstant=0.001  UdotUserProvided=0
  Suspension Front : Subsystem  mask(Suspension with Heave, Roll, and Ackerman Steering){zHeave=vehdata.SuspF.Heave.Height, kHeave=vehdata.SuspF.Heave.Stiffness, dHeave=vehdata.SuspF.Heave.Damping, xEqHeave=vehdata.SuspF.Heave.EqPos, zRoll=vehdata.SuspF.Roll.Height, kRoll=vehdata.SuspF.Roll.Stiffness, dRoll=vehdata.SuspF.Roll.Damping, aEqRoll=vehdata.SuspF.Roll.EqPos, mUnsprungMass=vehdata.SuspF.UnsprungMass.Mass, JUnsprungMass=vehdata.SuspF.UnsprungMass.Inertia, zUnsprungMass=vehdata.SuspF.UnsprungMass.Height, rUnsprungMass=vehdata.SuspF.UnsprungMass.Radius, lUnsprungMass=vehdata.SuspF.UnsprungMass.Length, zHub=vehdata.SuspF.Hub.Height, yTrack=vehdata.SuspF.Track, wheelbase=sum(abs(vehdata.Body.RA-vehdata.Body.FA)), steerRatio=vehdata.SuspF.SteerRatio}
      mask prompts: zHeave "Height (m)"; kHeave "Stiffness (N/m)"; dHeave "Damping (N/(m/s))"; xEqHeave "Equilibrium Position (m)"; zRoll "Height (m)"; kRoll "Stiffness (N*m/rad)"; dRoll "Damping (N*m/(rad/s)"; aEqRoll "Equilibrium Position (rad)"; mUnsprungMass "Mass (kg)"; JUnsprungMass "Inertia (kg*m^2)"; zUnsprungMass "Height (m)"; rUnsprungMass "Radius (m)"; lUnsprungMass "Length (m)"; zHub "Wheel Center Height (m)"; yTrack "Track Width (m)"; steerRatio "Steering Ratio"
      mask help: Models a suspension with heave and roll degrees of freedom for a single axle, with Ackermann steering. All heights are measured relative to the bottom of the wheels.
      settings: PortSchema="{\"entries\":[{\"content\":{\"sides\":[{\"content\":{\"connectorIds\":[\"LConn1\"]},\"type\":\"ConnectorPlacement.EquallySpacedRectSide\",\"uuid\":\"0af81f34-82de-4f02-a8a7-ec45be82faea\"},{\"content\":{\"connectorIds\":[\"In1\"],\"side\":\"RIGHT\"},\"type\":\"ConnectorPlacement.EquallySpacedRectSide\",\"uuid\":\"9bc48957-2707-4e2f-b988-a5743aaf8f58\"},{\"content\":{\"connectorIds\":[\"LConn2\"],\"side\":\"TOP\"},\"type\":\"ConnectorPlacement.EquallySpacedRectSide\",\"uuid\":\"08055243-2fee-46c8-8a4b-df5231c2978e\"},{\"content\":{\"connectorIds\":[\"RConn1\"],\"side\":\"BOTTOM\"},\"type\":\"ConnectorPlacement.EquallySpacedRectSide\",\"uuid\":\"745b1e5c-9113-4e99-a394-3eadcd3cd6f8\"}]},\"type\":\"ConnectorPlacement.EquallySpacedConnector\",\"uuid\":\"5011d399-f081-425d-a1fb-c00f3859766f\"}],\"packageUris\":[\"http://schema.mathworks.com/mf0/Connector/R2020b\"],\"version\":\"1.0\"}"
      mask DialogControl cont_heave_roll Prompt: Heave, Roll
      mask DialogControl group_heave Prompt: Heave
      mask DialogControl group_roll Prompt: Roll
      mask DialogControl cont_unsprung_mass Prompt: Unsprung Mass
      mask DialogControl cont_wheels_steering Prompt: Wheels, Steering
  Suspension Rear : Subsystem  mask(Suspension with Heave, Roll,){zHeave=vehdata.SuspR.Heave.Height, kHeave=vehdata.SuspR.Heave.Stiffness, dHeave=vehdata.SuspR.Heave.Damping, xEqHeave=vehdata.SuspR.Heave.EqPos, zRoll=vehdata.SuspR.Roll.Height, kRoll=vehdata.SuspR.Roll.Stiffness, dRoll=vehdata.SuspR.Roll.Damping, aEqRoll=vehdata.SuspR.Roll.EqPos, mUnsprungMass=vehdata.SuspR.UnsprungMass.Mass, JUnsprungMass=vehdata.SuspR.UnsprungMass.Inertia, zUnsprungMass=vehdata.SuspR.UnsprungMass.Height, rUnsprungMass=vehdata.SuspR.UnsprungMass.Radius, lUnsprungMass=vehdata.SuspR.UnsprungMass.Length, zHub=vehdata.SuspR.Hub.Height, yTrack=vehdata.SuspR.Track}
      mask prompts: zHeave "Height (m)"; kHeave "Stiffness (N/m)"; dHeave "Damping (N/(m/s))"; xEqHeave "Equilibrium Position (m)"; zRoll "Height (m)"; kRoll "Stiffness (N*m/rad)"; dRoll "Damping (N*m/(rad/s)"; aEqRoll "Equilibrium Position (rad)"; mUnsprungMass "Mass (kg)"; JUnsprungMass "Inertia (kg*m^2)"; zUnsprungMass "Height (m)"; rUnsprungMass "Radius (m)"; lUnsprungMass "Length (m)"; zHub "Wheel Center Height (m)"; yTrack "Track Width (m)"
      mask help: Models a suspension with heave and roll degrees of freedom for a single axle. All heights are measured relative to the bottom of the wheels.
      settings: PortSchema="{\"entries\":[{\"content\":{\"sides\":[{\"content\":{\"connectorIds\":[\"LConn1\"]},\"type\":\"ConnectorPlacement.EquallySpacedRectSide\",\"uuid\":\"0af81f34-82de-4f02-a8a7-ec45be82faea\"},{\"content\":{\"connectorIds\":[],\"side\":\"RIGHT\"},\"type\":\"ConnectorPlacement.EquallySpacedRectSide\",\"uuid\":\"9bc48957-2707-4e2f-b988-a5743aaf8f58\"},{\"content\":{\"connectorIds\":[\"LConn2\"],\"side\":\"TOP\"},\"type\":\"ConnectorPlacement.EquallySpacedRectSide\",\"uuid\":\"08055243-2fee-46c8-8a4b-df5231c2978e\"},{\"content\":{\"connectorIds\":[\"RConn1\"],\"side\":\"BOTTOM\"},\"type\":\"ConnectorPlacement.EquallySpacedRectSide\",\"uuid\":\"3fad50e5-0b96-4492-ad18-fd370deae0ca\"}]},\"type\":\"ConnectorPlacement.EquallySpacedConnector\",\"uuid\":\"5011d399-f081-425d-a1fb-c00f3859766f\"}],\"packageUris\":[\"http://schema.mathworks.com/mf0/Connector/R2020b\"],\"version\":\"1.0\"}"
      mask DialogControl cont_heave_roll Prompt: Heave, Roll
      mask DialogControl group_heave Prompt: Heave
      mask DialogControl group_roll Prompt: Roll
      mask DialogControl cont_unsprung_mass Prompt: Unsprung Mass
      mask DialogControl cont_wheels Prompt: Wheels
  Transform Scene : sm_lib/Frames and Transforms/Rigid Transform  RotationMethod=RotationSequence  FollAlignAxisA=+X  BaseAlignAxisA=+Y  FollAlignAxisB=+Y  BaseAlignAxisB=+Z  RotationStandardAxis=+Y  RotationAngle=0  RotationAngleUnits=deg  RotationArbitraryAxis=[0 0 1]  RotationSequenceAxes=FollowerAxes  RotationSequence=ZYX  RotationSequenceAngles=[SceneData.Reference.yaw SceneData.Reference.pitch SceneData.Reference.roll]  RotationSequenceAnglesUnits=rad  RotationMatrix=[1 0 0; 0 1 0; 0 0 1]  Quaternion=[1 0 0 0]  TranslationMethod=None  TranslationCartesianOffset=[0 0 0]  TranslationCartesianOffsetUnits=m  TranslationStandardAxis=+Z  TranslationStandardOffset=0  TranslationStandardOffsetUnits=m  TranslationROffset=0  TranslationROffsetUnits=m  TranslationThetaOffset=0  TranslationThetaOffsetUnits=deg  TranslationZOffset=0  TranslationZOffsetUnits=m
  Wheel FL : sm_vehicle_utilities_lib/Tire G  popup_leftright=Left  tire_param=vehdata.TireDataF.param  rim_mass=vehdata.RimF.Mass  rim_inertia=vehdata.RimF.Inertia
  Wheel FR : sm_vehicle_utilities_lib/Tire G  popup_leftright=Right  tire_param=vehdata.TireDataF.param  rim_mass=vehdata.RimF.Mass  rim_inertia=vehdata.RimF.Inertia
  Wheel RL : sm_vehicle_utilities_lib/Tire G  popup_leftright=Left  tire_param=vehdata.TireDataR.param  rim_mass=vehdata.RimR.Mass  rim_inertia=vehdata.RimR.Inertia
  Wheel RR : sm_vehicle_utilities_lib/Tire G  popup_leftright=Right  tire_param=vehdata.TireDataR.param  rim_mass=vehdata.RimR.Mass  rim_inertia=vehdata.RimR.Inertia
  World : Subsystem
  Out Bus Element9 : Outport  PortName=m  Element=Body
  Out Bus Element : Outport  PortName=m  Element=TireFL
  Out Bus Element1 : Outport  PortName=m  Element=TireFR
  Out Bus Element2 : Outport  PortName=m  Element=TireRL
  Out Bus Element3 : Outport  PortName=m  Element=TireRR
  Out Bus Element4 : Outport  PortName=m  Element=World
  wires:
  Wheel FL/1 -> [FL]
  Wheel RL/1 -> [RL]
  Wheel RR/1 -> [RR]
  Wheel FR/1 -> [FR]
  Bus Element In4/1 -> Suspension Front/1(s)
  Bus Element In/1 -> Simulink-PS Converter/1
  PS-Simulink Converter/1 -> [wFR]
  Bus Element In1/1 -> Simulink-PS Converter1/1
  PS-Simulink Converter1/1 -> [wRR]
  Bus Element In2/1 -> Simulink-PS Converter2/1
  PS-Simulink Converter2/1 -> [wRL]
  Bus Element In3/1 -> Simulink-PS Converter3/1
  PS-Simulink Converter3/1 -> [wFL]
  Body/1(m) -> Out Bus Element9/1
  [wFL] -> Outputs/1(wFL)
  [FL] -> Outputs/2(TFL)
  Outputs/1(FL) -> Out Bus Element/1
  [wFR] -> Outputs/3(wFR)
  [FR] -> Outputs/4(TFR)
  [wRL] -> Outputs/5(wRL)
  [RL] -> Outputs/6(TRL)
  [wRR] -> Outputs/7(wRR)
  [RR] -> Outputs/8(TRR)
  Outputs/2(FR) -> Out Bus Element1/1
  Outputs/3(RL) -> Out Bus Element2/1
  Outputs/4(RR) -> Out Bus Element3/1
  Body to World/1 -> Out Bus Element4/1
  connections:
  Body to World/LConn1 -- Grid Surface/LConn1 -- Transform Scene/LConn1 -- World/RConn1
  Body/LConn1 -- Suspension Rear/LConn1
  Wheel FR/LConn2 -- Revolute FR/RConn1
  Suspension Front/RConn1 -- Revolute FR/LConn1
  Suspension Front/LConn2 -- Revolute FL/LConn1
  Suspension Rear/LConn2 -- Revolute RL/LConn1
  Revolute RR/LConn1 -- Suspension Rear/RConn1
  Wheel RL/LConn2 -- Revolute RL/RConn1
  Camera Frames/RConn1 -- Body to World/RConn1 -- Body/RConn2
  Wheel FL/LConn2 -- Revolute FL/RConn1
  Wheel RR/LConn2 -- Revolute RR/RConn1
  Suspension Front/LConn1 -- Body/RConn1
  Revolute FR/RConn2 -- PS-Simulink Converter/LConn1
  Simulink-PS Converter/RConn1 -- Revolute FR/LConn2
  Simulink-PS Converter1/RConn1 -- Revolute RR/LConn2
  PS-Simulink Converter1/LConn1 -- Revolute RR/RConn2
  Simulink-PS Converter2/RConn1 -- Revolute RL/LConn2
  PS-Simulink Converter2/LConn1 -- Revolute RL/RConn2
  Simulink-PS Converter3/RConn1 -- Revolute FL/LConn2
  PS-Simulink Converter3/LConn1 -- Revolute FL/RConn2
  Scene/RConn1 -- Transform Scene/RConn1
  Wheel FL/LConn3 -- Grid Surface/RConn1 -- Connection Label4/LConn1
  Connection Label1/LConn1 -- Wheel FR/LConn3
  Connection Label2/LConn1 -- Wheel RR/LConn3
  Connection Label3/LConn1 -- Wheel RL/LConn3

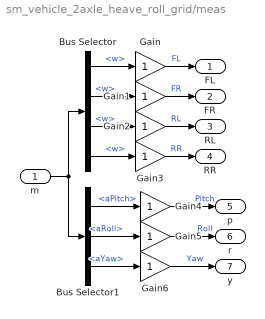
== system sm_vehicle_2axle_heave_roll_grid/meas ==
  m : Inport
  Bus Selector : BusSelector  OutputSignals=TireFL.w,TireFR.w,TireRL.w,TireRR.w
  Bus Selector1 : BusSelector  OutputSignals=Body.aPitch,Body.aRoll,World.aYaw
  Gain{,1..6} (7 alike) : Gain
  FL : Outport
  FR : Outport  Port=2
  RL : Outport  Port=3
  RR : Outport  Port=4
  p : Outport  Port=5
  r : Outport  Port=6
  y : Outport  Port=7
  wires:
  Bus Selector/4 -> Gain3/1  "<w>"
  Bus Selector/2 -> Gain1/1  "<w>"
  Bus Selector/3 -> Gain2/1  "<w>"
  Bus Selector/1 -> Gain/1  "<w>"
  m/1 -> Bus Selector/1, Bus Selector1/1
  Gain3/1 -> RR/1  "RR"
  Gain/1 -> FL/1  "FL"
  Gain1/1 -> FR/1  "FR"
  Gain2/1 -> RL/1  "RL"
  Bus Selector1/1 -> Gain4/1  "<aPitch>"
  Bus Selector1/2 -> Gain5/1  "<aRoll>"
  Bus Selector1/3 -> Gain6/1  "<aYaw>"
  Gain6/1 -> y/1  "Yaw"
  Gain5/1 -> r/1  "Roll"
  Gain4/1 -> p/1  "Pitch"

== system sm_vehicle_2axle_heave_roll_grid/Driver Input/No Steer ==
  Bus Creator : BusCreator  Inputs=5
  Constant{,1..4} (5 alike) : Constant  Value=0
  Drv : Outport
  wires:
  Constant/1 -> Bus Creator/1  "sWhl"
  Constant3/1 -> Bus Creator/4  "trqRL"
  Constant2/1 -> Bus Creator/3  "trqFR"
  Constant4/1 -> Bus Creator/5  "trqRR"
  Bus Creator/1 -> Drv/1
  Constant1/1 -> Bus Creator/2  "trqFL"

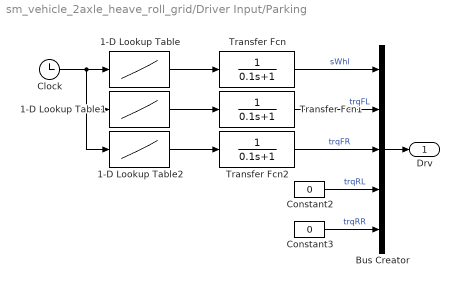
== system sm_vehicle_2axle_heave_roll_grid/Driver Input/Parking ==
  1-D Lookup Table : Lookup_n-D  NumberOfTableDimensions=1  BreakpointsForDimension1=Maneuver.Parking.Steer.tvec  Table=Maneuver.Parking.Steer.aSteerWheel  InternalRulePriority=Speed  RndMeth=Simplest
  1-D Lookup Table1 : Lookup_n-D  NumberOfTableDimensions=1  BreakpointsForDimension1=Maneuver.Parking.Wheel.tvec  Table=Maneuver.Parking.Wheel.trqFL  InternalRulePriority=Speed  RndMeth=Simplest
  1-D Lookup Table2 : Lookup_n-D  NumberOfTableDimensions=1  BreakpointsForDimension1=Maneuver.Parking.Wheel.tvec  Table=Maneuver.Parking.Wheel.trqFR  RemoveProtectionInput=on  InternalRulePriority=Speed  RndMeth=Simplest
  Bus Creator : BusCreator  Inputs=5
  Clock : Clock
  Constant2 : Constant  Value=0
  Constant3 : Constant  Value=0
  Transfer Fcn : TransferFcn  Denominator=[0.1 1]
  Transfer Fcn1 : TransferFcn  Denominator=[0.1 1]
  Transfer Fcn2 : TransferFcn  Denominator=[0.1 1]
  Drv : Outport
  wires:
  Clock/1 -> 1-D Lookup Table2/1, 1-D Lookup Table1/1, 1-D Lookup Table/1
  1-D Lookup Table/1 -> Transfer Fcn/1
  Constant2/1 -> Bus Creator/4  "trqRL"
  Transfer Fcn2/1 -> Bus Creator/3  "trqFR"
  Constant3/1 -> Bus Creator/5  "trqRR"
  Bus Creator/1 -> Drv/1
  Transfer Fcn1/1 -> Bus Creator/2  "trqFL"
  Transfer Fcn/1 -> Bus Creator/1  "sWhl"
  1-D Lookup Table1/1 -> Transfer Fcn1/1
  1-D Lookup Table2/1 -> Transfer Fcn2/1

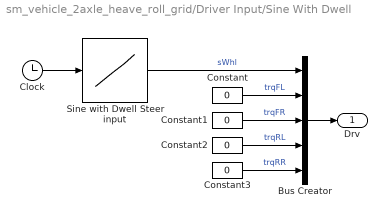
== system sm_vehicle_2axle_heave_roll_grid/Driver Input/Sine With Dwell ==
  Bus Creator : BusCreator  Inputs=5
  Clock : Clock
  Constant{,1..3} (4 alike) : Constant  Value=0
  Sine with Dwell Steer input : Lookup  InputValues=Maneuver.SineWithDwell.tvec  Table=Maneuver.SineWithDwell.aStrWheel  SaturateOnIntegerOverflow=off
  Drv : Outport
  wires:
  Clock/1 -> Sine with Dwell Steer input/1
  Sine with Dwell Steer input/1 -> Bus Creator/1  "sWhl"
  Constant/1 -> Bus Creator/2  "trqFL"
  Constant1/1 -> Bus Creator/3  "trqFR"
  Constant2/1 -> Bus Creator/4  "trqRL"
  Constant3/1 -> Bus Creator/5  "trqRR"
  Bus Creator/1 -> Drv/1

== system sm_vehicle_2axle_heave_roll_grid/Driver Input/Slalom ==
  Bus Creator : BusCreator  Inputs=5
  Constant : Constant  Value=38
  Constant1 : Constant  Value=38
  Constant2 : Constant  Value=0
  Constant3 : Constant  Value=0
  Sine Wave : Sin  Amplitude=20*(pi/180)  Frequency=4*pi/10  Phase=pi/2+0.01  SampleTime=0
  Drv : Outport
  wires:
  Sine Wave/1 -> Bus Creator/1  "sWhl"
  Constant/1 -> Bus Creator/2  "trqFL"
  Constant1/1 -> Bus Creator/3  "trqFR"
  Constant2/1 -> Bus Creator/4  "trqRL"
  Constant3/1 -> Bus Creator/5  "trqRR"
  Bus Creator/1 -> Drv/1

== system sm_vehicle_2axle_heave_roll_grid/Driver Input/Step Steer ==
  Bus Creator : BusCreator  Inputs=5
  Constant{,1..3} (4 alike) : Constant  Value=0
  Step Steer input : Step  Time=3  After=160*pi/180  SampleTime=0
  Drv : Outport
  wires:
  Step Steer input/1 -> Bus Creator/1  "sWhl"
  Constant2/1 -> Bus Creator/4  "trqRL"
  Constant1/1 -> Bus Creator/3  "trqFR"
  Constant3/1 -> Bus Creator/5  "trqRR"
  Bus Creator/1 -> Drv/1
  Constant/1 -> Bus Creator/2  "trqFL"
